simulink model "class_5_simulink"  (R2023b)
settings: Solver=VariableStepAuto  StartTime=0.0  StopTime=40  RelTol=1e-3
values from neighbouring files (symbols this model uses):
  denp = [3 1]    [class_5.m]
  h = 6.5    [class_5.m]
  hd = h/Ts    (= 26)    [class_5.m]
  I = eye(size(A))    [class_5.m]
  K = 6.7*(-A)    [class_5.m]
  Kd = Ad    [class_5.m]
  kr = (c*((B*K-A)^(-1))*B)^(-1)    [class_5.m]
  krd = (Cd*((Bd*Kd-Ad)^(-1))*Bd)^(-1)    [class_5.m]
  nump = [0 2]    [class_5.m]
  s = tf('s')    [class_5.m]
  Ts = 0.25    [class_5.m]
  zo = tf('z',Ts)    [class_5.m]
undefined symbols (not defined in the file or in its folder): A, Ad, B, Bd
libraries: cstblocks x21
settings Model: Creator=klysm  LastModifiedBy=klysm

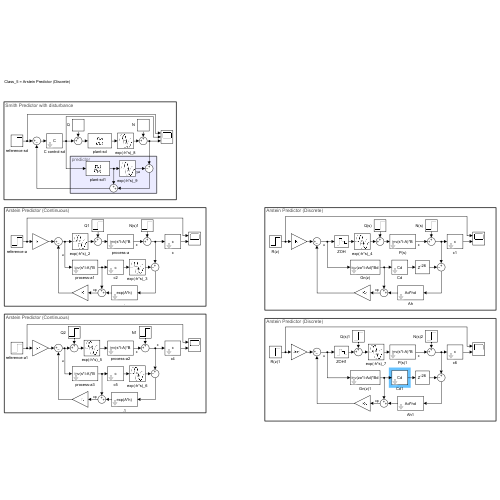
[thumbnail: Simulink's stored preview of the top-level diagram]
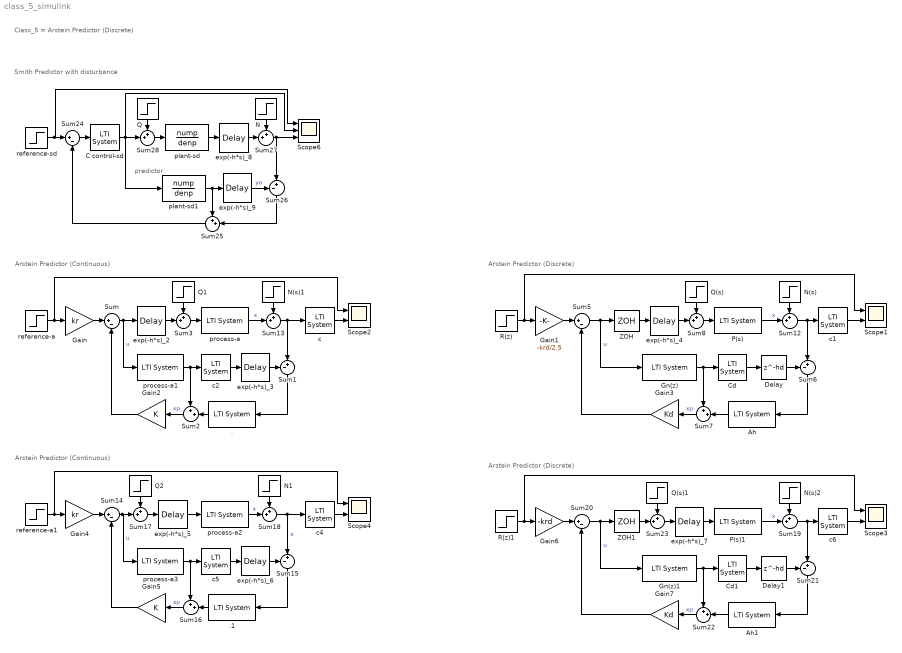
== system class_5_simulink ==
  note: Class_5 = Arstein Predictor (Discrete)
  note: Arstein Predictor (Discrete)
  note: Arstein Predictor (Continuous)
  note: Arstein Predictor (Continuous)
  note: Arstein Predictor (Discrete)
  note: Smith Predictor with disturbance
  note: predictor
  . : cstblocks/LTI System  sys=exp(A*h)  IC=[]  PadeOrder=0
  .1 : cstblocks/LTI System  sys=exp(A*h)  IC=[]  PadeOrder=0
  Ah : cstblocks/LTI System  sys=Ad^hd  IC=[]  PadeOrder=0
  Ah1 : cstblocks/LTI System  sys=Ad^hd  IC=[]  PadeOrder=0
  C control-sd : cstblocks/LTI System  sys=C  IC=[]  PadeOrder=0
  Cd : cstblocks/LTI System  sys=Cd  IC=[]  PadeOrder=0
  Cd1 : cstblocks/LTI System  sys=Cd  IC=[]  PadeOrder=0
  Delay : Delay  DelayLength=hd
  Delay1 : Delay  DelayLength=hd
  Gain : Gain  Gain=kr
  Gain1 : Gain  Gain=-krd/2.5
  Gain2 : Gain  Gain=K
  Gain3 : Gain  Gain=Kd
  Gain4 : Gain  Gain=kr
  Gain5 : Gain  Gain=K
  Gain6 : Gain  Gain=-krd
  Gain7 : Gain  Gain=Kd
  Gn(z) : cstblocks/LTI System  sys=inv(zo*I-Ad)*Bd  IC=[]  PadeOrder=0
  Gn(z)1 : cstblocks/LTI System  sys=inv(zo*I-Ad)*Bd  IC=[]  PadeOrder=0
  N : Step  Time=20  After=0.2  SampleTime=0
  N(s) : Step  Time=20  After=0.2  SampleTime=0
  N(s)1 : Step  Time=20  After=0.2  SampleTime=0
  N(s)2 : Step  Time=20  After=0.2  SampleTime=0
  N1 : Step  Time=20  After=0.2  SampleTime=0
  P(s) : cstblocks/LTI System  sys=inv(s*I-A)*B  IC=[]  PadeOrder=0
  P(s)1 : cstblocks/LTI System  sys=inv(s*I-A)*B  IC=[]  PadeOrder=0
  Q : Step  Time=10  After=0.2  SampleTime=0
  Q(s) : Step  Time=10  After=0.2  SampleTime=0
  Q(s)1 : Step  Time=10  After=0.2  SampleTime=0
  Q1 : Step  Time=10  After=0.2  SampleTime=0
  Q2 : Step  Time=10  After=0.2  SampleTime=0
  R(z) : Step  Time=0  SampleTime=Ts
  R(z)1 : Step  Time=0  SampleTime=Ts
  Scope{1..4} (4 alike) : Scope  NumInputPorts=2
  Scope6 : Scope  NumInputPorts=3
  Sum{,5,14,20,24} (5 alike) : Sum  Inputs=|+-
  Sum{1,6,15,21,26} (5 alike) : Sum  Inputs=-+|
  Sum{2..3,7..8,12..13,16..19,22..23,25,27..28} (15 alike) : Sum  Inputs=++|
  ZOH : ZeroOrderHold  SampleTime=-1
  ZOH1 : ZeroOrderHold  SampleTime=-1
  c{,1..2,4..6} (6 alike) : cstblocks/LTI System  sys=c  IC=[]  PadeOrder=0
  exp(-h*s)_{2..9} (8 alike) : TransportDelay  DelayTime=h
  plant-sd : TransferFcn  Numerator=nump  Denominator=denp
  plant-sd1 : TransferFcn  Numerator=nump  Denominator=denp
  process-a{,1..3} (4 alike) : cstblocks/LTI System  sys=inv(s*I-A)*B  IC=[]  PadeOrder=0
  reference-a : Step  Time=0  SampleTime=0
  reference-a1 : Step  Time=0  SampleTime=0
  reference-sd : Step  Time=0  SampleTime=0
  wires:
  c1/1 -> Scope1/2
  Gain3/1 -> Sum5/2
  Sum8/1 -> P(s)/1
  Sum7/1 -> Gain3/1  "xp"
  Sum6/1 -> Ah/1
  Ah/1 -> Sum7/2
  R(z)/1 -> Scope1/1, Gain1/1
  Delay/1 -> Sum6/1
  Q(s)/1 -> Sum8/1
  Gn(z)/1 -> Cd/1, Sum7/1
  Gain1/1 -> Sum5/1
  exp(-h*s)_4/1 -> Sum8/2
  P(s)/1 -> Sum12/2  "x"
  Sum12/1 -> Sum6/2, c1/1
  N(s)/1 -> Sum12/1
  Sum5/1 -> ZOH/1, Gn(z)/1  "u"
  c/1 -> Scope2/2
  exp(-h*s)_3/1 -> Sum1/1
  process-a1/1 -> c2/1, Sum2/1
  Gain/1 -> Sum/1
  reference-a/1 -> Scope2/1, Gain/1
  exp(-h*s)_2/1 -> Sum3/2
  Sum1/1 -> ./1
  Sum/1 -> process-a1/1, exp(-h*s)_2/1  "u"
  ./1 -> Sum2/2
  Gain2/1 -> Sum/2
  Sum2/1 -> Gain2/1  "xp"
  Sum3/1 -> process-a/1
  c2/1 -> exp(-h*s)_3/1
  Q1/1 -> Sum3/1
  Cd/1 -> Delay/1
  process-a/1 -> Sum13/2  "x"
  Sum13/1 -> Sum1/2, c/1
  N(s)1/1 -> Sum13/1
  ZOH/1 -> exp(-h*s)_4/1
  Sum17/1 -> exp(-h*s)_5/1
  .1/1 -> Sum16/2
  exp(-h*s)_5/1 -> process-a2/1
  c4/1 -> Scope4/2
  Sum14/1 -> Sum17/2, process-a3/1  "u"
  Sum16/1 -> Gain5/1  "xp"
  exp(-h*s)_6/1 -> Sum15/1
  process-a3/1 -> c5/1, Sum16/1
  N1/1 -> Sum18/1
  c5/1 -> exp(-h*s)_6/1
  Gain5/1 -> Sum14/2
  reference-a1/1 -> Scope4/1, Gain4/1
  Sum15/1 -> .1/1
  Sum18/1 -> c4/1, Sum15/2  "x"
  Q2/1 -> Sum17/1
  process-a2/1 -> Sum18/2  "x"
  Gain4/1 -> Sum14/1
  P(s)1/1 -> Sum19/2  "x"
  ZOH1/1 -> Sum23/2
  N(s)2/1 -> Sum19/1
  Delay1/1 -> Sum21/1
  Sum19/1 -> Sum21/2, c6/1
  Cd1/1 -> Delay1/1
  R(z)1/1 -> Scope3/1, Gain6/1
  Ah1/1 -> Sum22/2
  Sum20/1 -> ZOH1/1, Gn(z)1/1  "u"
  Gn(z)1/1 -> Cd1/1, Sum22/1
  Gain6/1 -> Sum20/1
  exp(-h*s)_7/1 -> P(s)1/1
  Gain7/1 -> Sum20/2
  Sum22/1 -> Gain7/1  "xp"
  Sum21/1 -> Ah1/1
  c6/1 -> Scope3/2
  Sum23/1 -> exp(-h*s)_7/1
  Q(s)1/1 -> Sum23/1
  Sum24/1 -> C control-sd/1
  Sum26/1 -> Sum25/2
  Sum25/1 -> Sum24/2
  exp(-h*s)_8/1 -> Sum27/2
  C control-sd/1 -> Sum28/2, Scope6/2, plant-sd1/1
  plant-sd1/1 -> Sum25/1, exp(-h*s)_9/1
  exp(-h*s)_9/1 -> Sum26/1  "ya"
  plant-sd/1 -> exp(-h*s)_8/1
  Sum27/1 -> Scope6/3, Sum26/2
  Sum28/1 -> plant-sd/1
  reference-sd/1 -> Scope6/1, Sum24/1
  N/1 -> Sum27/1
  Q/1 -> Sum28/1
